simulink subsystem "subsystem_controller_simplified"  (R2022a)
settings: Solver=VariableStepAuto  StartTime=0.0  StopTime=10.0  RelTol=1e-3
libraries: neuromorphic_blocks x22
settings Model: Creator=chris  LastModifiedBy=chris

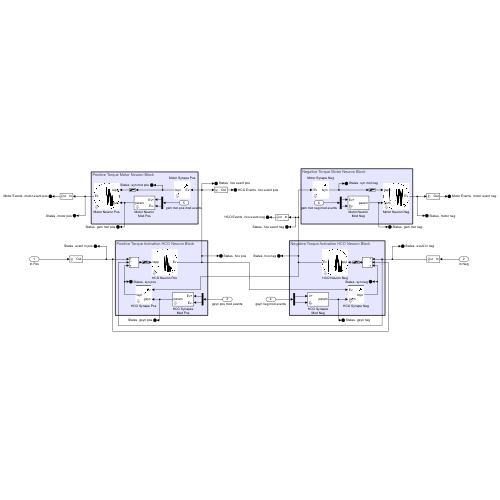
[thumbnail: Simulink's stored preview of the top-level diagram]
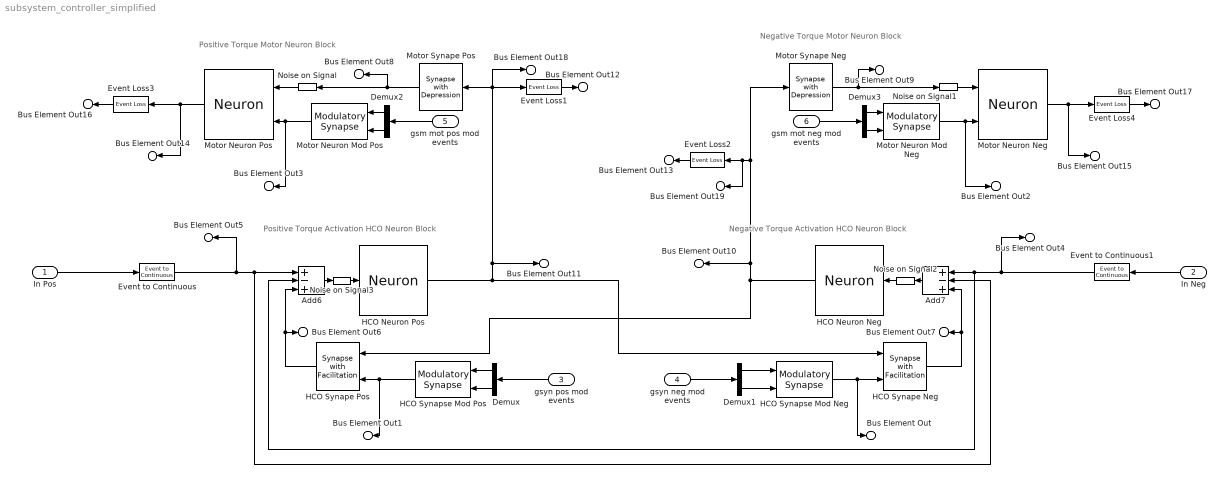
== system subsystem_controller_simplified ==
  note: Positive Torque Motor Neuron Block
  note: Negative Torque Activation HCO Neuron Block
  note: Positive Torque Activation HCO Neuron Block
  note: Negative Torque Motor Neuron Block
  In Pos : Inport
  In Neg : Inport  Port=2
  gsyn pos mod events : Inport  Port=3
  gsyn neg mod events : Inport  Port=4
  gsm mot pos mod events : Inport  Port=5
  gsm mot neg mod events : Inport  Port=6
  Add6 : Sum  Inputs=+-+
  Add7 : Sum  Inputs=+-+
  Demux{,1..3} (4 alike) : Demux  Outputs=2
  Event Loss{1..4} (4 alike) : neuromorphic_blocks/Events Transmission Blocks/Event Loss  loss_prob=prob_event_loss  seed=-1  seed_mem=randi([0, 100000])
      settings: SourceProductName=Neuromorphic Toolbox
  Event to Continuous : neuromorphic_blocks/Events Transmission Blocks/Event to Continuous  gain=0.2
      settings: SourceProductName=Neuromorphic Toolbox
  Event to Continuous1 : neuromorphic_blocks/Events Transmission Blocks/Event to Continuous  gain=0.2
      settings: SourceProductName=Neuromorphic Toolbox
  HCO Neuron Neg : neuromorphic_blocks/Neural Blocks/Neuron  gfm_source=Internal  gfm=3  gsp_source=Internal  gsp=6  gsm_source=Internal  gsm=3  gup_source=Internal  gup=5  gum_source=Internal  gum=2  dfm=0  dsp=0.5  dsm=-0.5  dup=-0.5  dum=-1.0  mfm=1  msp=1  msm=1  mup=1  mum=1  timescale=timescale  rel_membrane=0.1  rel_fast=0.1  rel_slow=4  rel_ultraslow=200  Iapp_base=0.2  V0=-1.2  tresh=0.0  output=Events
      settings: SourceProductName=Neuromorphic Toolbox
  HCO Neuron Pos : neuromorphic_blocks/Neural Blocks/Neuron  gfm_source=Internal  gfm=3  gsp_source=Internal  gsp=6  gsm_source=Internal  gsm=3  gup_source=Internal  gup=5  gum_source=Internal  gum=2  dfm=0  dsp=0.5  dsm=-0.5  dup=-0.5  dum=-1.0  mfm=1  msp=1  msm=1  mup=1  mum=1  timescale=timescale  rel_membrane=0.1  rel_fast=0.1  rel_slow=4  rel_ultraslow=200  Iapp_base=0.2  V0=-1.2  tresh=0  output=Events
      settings: SourceProductName=Neuromorphic Toolbox
  HCO Synape Neg : neuromorphic_blocks/Neural Blocks/Synapse with Facilitation  gsyn_source=External  gsyn=-2  dsyn=10  msyn=20  timescale=timescale  rel_timescale=10  input=Events  gsyn_in=0  dsyn_in=0  msyn_in=1
      settings: SourceProductName=Neuromorphic Toolbox
  HCO Synape Pos : neuromorphic_blocks/Neural Blocks/Synapse with Facilitation  gsyn_source=External  gsyn=-2  dsyn=10  msyn=20  timescale=timescale  rel_timescale=10  input=Events  gsyn_in=0  dsyn_in=0  msyn_in=1
      settings: SourceProductName=Neuromorphic Toolbox
  HCO Synapse Mod Neg : neuromorphic_blocks/Neural Blocks/Modulatory Synapse  base_val=base_gsyn  gsyn_pos_source=Internal  gsyn_pos=mod_strength_gsyn  gsyn_neg_source=Internal  gsyn_neg=mod_strength_gsyn  timescale=timescale  rel_timescale=rel_mod  input=Events  dsyn_pos=10  dsyn_neg=10  msyn_pos=20  msyn_neg=20
      settings: SourceProductName=Neuromorphic Toolbox
  HCO Synapse Mod Pos : neuromorphic_blocks/Neural Blocks/Modulatory Synapse  base_val=base_gsyn  gsyn_pos_source=Internal  gsyn_pos=mod_strength_gsyn  gsyn_neg_source=Internal  gsyn_neg=mod_strength_gsyn  timescale=timescale  rel_timescale=rel_mod  input=Events  dsyn_pos=10  dsyn_neg=10  msyn_pos=20  msyn_neg=20
      settings: SourceProductName=Neuromorphic Toolbox
  Motor Neuron Mod Neg : neuromorphic_blocks/Neural Blocks/Modulatory Synapse  base_val=base_gsm  gsyn_pos_source=Internal  gsyn_pos=mod_strength_gsm  gsyn_neg_source=Internal  gsyn_neg=mod_strength_gsm  timescale=timescale  rel_timescale=rel_mod  input=Events  dsyn_pos=10  dsyn_neg=10  msyn_pos=20  msyn_neg=20
      settings: SourceProductName=Neuromorphic Toolbox
  Motor Neuron Mod Pos : neuromorphic_blocks/Neural Blocks/Modulatory Synapse  base_val=base_gsm  gsyn_pos_source=Internal  gsyn_pos=mod_strength_gsm  gsyn_neg_source=Internal  gsyn_neg=mod_strength_gsm  timescale=timescale  rel_timescale=rel_mod  input=Events  dsyn_pos=10  dsyn_neg=10  msyn_pos=20  msyn_neg=20
      settings: SourceProductName=Neuromorphic Toolbox
  Motor Neuron Neg : neuromorphic_blocks/Neural Blocks/Neuron  gfm_source=Internal  gfm=3  gsp_source=Internal  gsp=6  gsm_source=External  gsm=2.3  gup_source=Internal  gup=5  gum_source=Internal  gum=2  dfm=0  dsp=0.5  dsm=-0.5  dup=-0.5  dum=-1.0  mfm=1  msp=1  msm=1  mup=1  mum=1  timescale=timescale  rel_membrane=0.1  rel_fast=0.1  rel_slow=4  rel_ultraslow=200  Iapp_base=-0.5  V0=-1.2  tresh=0  output=Events
      settings: SourceProductName=Neuromorphic Toolbox
  Motor Neuron Pos : neuromorphic_blocks/Neural Blocks/Neuron  gfm_source=Internal  gfm=3  gsp_source=Internal  gsp=6  gsm_source=External  gsm=2.3  gup_source=Internal  gup=5  gum_source=Internal  gum=2  dfm=0  dsp=0.5  dsm=-0.5  dup=-0.5  dum=-1.0  mfm=1  msp=1  msm=1  mup=1  mum=1  timescale=timescale  rel_membrane=0.1  rel_fast=0.1  rel_slow=4  rel_ultraslow=200  Iapp_base=-0.5  V0=-1.2  tresh=0  output=Events
      settings: SourceProductName=Neuromorphic Toolbox
  Motor Synape Neg : neuromorphic_blocks/Neural Blocks/Synapse with Depression  gsyn_source=Internal  gsyn=4  dsyn=10  msyn=20  dsyn_dep=15  msyn_dep=100  timescale=timescale  rel_facilitation=0  rel_depression=100  input=Events  gsyn_in=0  dsyn_in=0  msyn_in=1
      settings: SourceProductName=Neuromorphic Toolbox
  Motor Synape Pos : neuromorphic_blocks/Neural Blocks/Synapse with Depression  gsyn_source=Internal  gsyn=4  dsyn=10  msyn=20  dsyn_dep=15  msyn_dep=100  timescale=timescale  rel_facilitation=0  rel_depression=100  input=Events  gsyn_in=0  dsyn_in=0  msyn_in=1
      settings: SourceProductName=Neuromorphic Toolbox
  Noise on Signal{,1..3} (4 alike) : neuromorphic_blocks/Auxiliary Blocks/Noise on Signal  noise_pwr=noisePwr  timescale=timescale  rel_timescale=rel_noise  seed=-1  seed_mem=randi([0, 100000])
      settings: SourceProductName=NeurCont Toolbox
  Bus Element Out12 : Outport  PortName=HCO Events  Element=hco event pos
  Bus Element Out13 : Outport  PortName=HCO Events  Element=hco event neg
  Bus Element Out17 : Outport  Port=2  PortName=Motor Events  Element=motor event neg
  Bus Element Out16 : Outport  Port=2  PortName=Motor Events  Element=motor event pos
  Bus Element Out : Outport  Port=3  PortName=States  Element=gsyn neg
  Bus Element Out1 : Outport  Port=3  PortName=States  Element=gsyn pos
  Bus Element Out6 : Outport  Port=3  PortName=States  Element=syn pos
  Bus Element Out7 : Outport  Port=3  PortName=States  Element=syn neg
  Bus Element Out2 : Outport  Port=3  PortName=States  Element=gsm mot neg
  Bus Element Out4 : Outport  Port=3  PortName=States  Element=event in neg
  Bus Element Out9 : Outport  Port=3  PortName=States  Element=syn mot neg
  Bus Element Out15 : Outport  Port=3  PortName=States  Element=motor neg
  Bus Element Out3 : Outport  Port=3  PortName=States  Element=gsm mot pos
  Bus Element Out5 : Outport  Port=3  PortName=States  Element=event in pos
  Bus Element Out8 : Outport  Port=3  PortName=States  Element=syn mot pos
  Bus Element Out14 : Outport  Port=3  PortName=States  Element=motor pos
  Bus Element Out10 : Outport  Port=3  PortName=States  Element=hco neg
  Bus Element Out11 : Outport  Port=3  PortName=States  Element=hco pos
  Bus Element Out18 : Outport  Port=3  PortName=States  Element=hco event pos
  Bus Element Out19 : Outport  Port=3  PortName=States  Element=hco event neg
  wires:
  In Neg/1 -> Event to Continuous1/1
  Motor Synape Neg/1 -> Bus Element Out9/1, Noise on Signal1/1
  HCO Synapse Mod Pos/1 -> HCO Synape Pos/2, Bus Element Out1/1
  gsyn pos mod events/1 -> Demux/1
  HCO Synape Pos/1 -> Add6/3, Bus Element Out6/1
  Motor Synape Pos/1 -> Noise on Signal/1, Bus Element Out8/1
  In Pos/1 -> Event to Continuous/1
  Event to Continuous/1 -> Add7/2, Add6/1, Bus Element Out5/1
  gsyn neg mod events/1 -> Demux1/1
  Event to Continuous1/1 -> Add6/2, Add7/1, Bus Element Out4/1
  Motor Neuron Mod Neg/1 -> Bus Element Out2/1, Motor Neuron Neg/2
  HCO Synapse Mod Neg/1 -> Bus Element Out/1, HCO Synape Neg/2
  gsm mot pos mod events/1 -> Demux2/1
  gsm mot neg mod events/1 -> Demux3/1
  Motor Neuron Mod Pos/1 -> Motor Neuron Pos/2, Bus Element Out3/1
  HCO Synape Neg/1 -> Add7/3, Bus Element Out7/1
  Event Loss1/1 -> Bus Element Out12/1
  Event Loss2/1 -> Bus Element Out13/1
  Demux1/1 -> HCO Synapse Mod Neg/1
  Demux1/2 -> HCO Synapse Mod Neg/2
  Demux/1 -> HCO Synapse Mod Pos/1
  Demux/2 -> HCO Synapse Mod Pos/2
  Demux2/1 -> Motor Neuron Mod Pos/1
  Demux2/2 -> Motor Neuron Mod Pos/2
  Demux3/1 -> Motor Neuron Mod Neg/1
  Demux3/2 -> Motor Neuron Mod Neg/2
  Motor Neuron Pos/1 -> Bus Element Out14/1, Event Loss3/1
  Event Loss3/1 -> Bus Element Out16/1
  Motor Neuron Neg/1 -> Bus Element Out15/1, Event Loss4/1
  Event Loss4/1 -> Bus Element Out17/1
  Noise on Signal/1 -> Motor Neuron Pos/1
  Noise on Signal1/1 -> Motor Neuron Neg/1
  Noise on Signal2/1 -> HCO Neuron Neg/1
  Add7/1 -> Noise on Signal2/1
  Add6/1 -> Noise on Signal3/1
  Noise on Signal3/1 -> HCO Neuron Pos/1
  HCO Neuron Pos/1 -> Bus Element Out18/1, Event Loss1/1, Motor Synape Pos/1, Bus Element Out11/1, HCO Synape Neg/1
  HCO Neuron Neg/1 -> Bus Element Out19/1, Event Loss2/1, Motor Synape Neg/1, Bus Element Out10/1, HCO Synape Pos/1
